simulink model "Simulation_Steam_Governor"  (R2024b)
settings: Solver=VariableStepAuto  StartTime=0.0  StopTime=10.0  RelTol=1e-3
model workspace (MAT data in the model file):
  Cd = 3
  Fg = 39.24
  I = 4
  L = 1
  g = 9.81
  m = 4
settings Model: Creator=arthu  LastModifiedBy=arthu

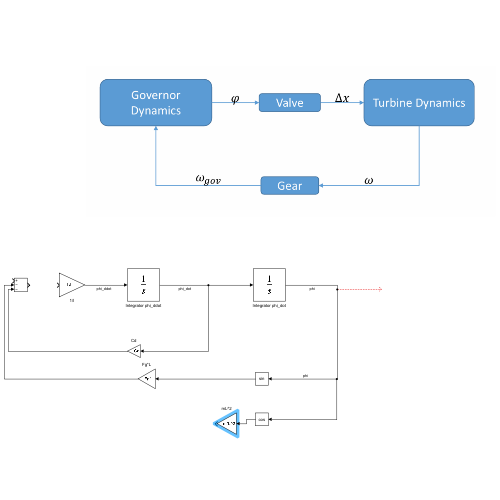
[thumbnail: Simulink's stored preview of the top-level diagram]
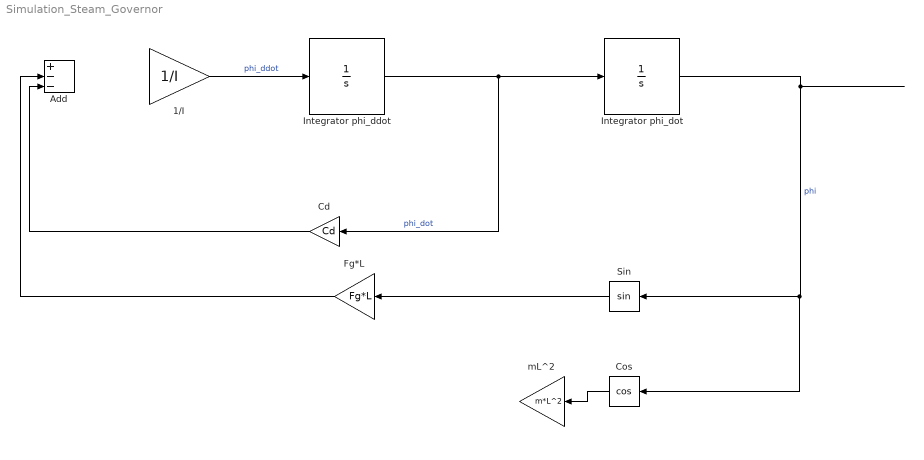
== system Simulation_Steam_Governor ==
  1/I : Gain  Gain=1/I
  Add : Sum  Inputs=+--
  Cd : Gain  Gain=Cd
  Cos : Trigonometry  Operator=cos
  Fg*L : Gain  Gain=Fg*L
  Integrator phi_ddot : Integrator
  Integrator phi_dot : Integrator
  Sin : Trigonometry
  mL^2 : Gain  Gain=m*L^2
  wires:
  Integrator phi_ddot/1 -> Cd/1, Integrator phi_dot/1  "phi_dot"
  Integrator phi_dot/1 -> Cos/1, Sin/1  "phi"
  1/I/1 -> Integrator phi_ddot/1  "phi_ddot"
  Cd/1 -> Add/3
  Fg*L/1 -> Add/2
  Sin/1 -> Fg*L/1
  Cos/1 -> mL^2/1
